simulink model "Assingment1_3K04_Part1_Group_7"  (R2017b)
settings: Solver=FixedStepAuto  StartTime=0.0  StopTime=3  FixedStep=1e-3  RelTol=1e-3  EnableMultiTasking=on
undefined symbols (not defined in the file): D10, D11, D12, D13, D2, D3, D4, D5, D6, D7, D8, D9, PTA0, PTA1, PTA2, PTB23, PTB9, PTC2, PTC3, PTC4, PTD0, PTD1, PTD2, PTD3
libraries: frdmk64flib x14
settings Model: ExtModeTrigDuration=5  Creator=howla_000  LastModifiedBy=gagiche
settings DataIOCC: LimitDataPoints=on  SaveFormat=Array
settings OptimizationCC: PassReuseOutputArgsAs=Individual arguments  MaxStackSize=64
settings DebuggingCC: UnderspecifiedInitializationDetection=Classic  MergeDetectMultiDrivingBlocksExec=none  SolverPrmCheckMsg=warning  ParameterTunabilityLossMsg=error  StateNameClashWarn=warning  SFUnexpectedBacktrackingDiag=warning  SFNoUnconditionalDefaultTransitionDiag=warning  SFExecutionAtInitializationDiag=none
settings HardwareCC: ProdBitPerPointer=32  ProdBitPerSizeT=32  ProdBitPerPtrDiffT=32  ProdLargestAtomicInteger=Long  ProdLargestAtomicFloat=Double  ProdWordSize=32  ProdHWDeviceType=ARM Compatible->ARM Cortex
settings ModelReferenceCC: PropagateSignalLabelsOutOfModel=off
settings SFSimCC: MATLABDynamicMemAlloc=off
settings RTWCC: SystemTargetFile=ert.tlc  HardwareBoard=NXP FRDM-K64F  TemplateMakefile=ert_default_tmf  GenerateReport=on  Toolchain=GNU Tools for ARM Embedded Processors  IncludeHyperlinkInReport=on  LaunchReport=on  GenerateTraceInfo=on  GenerateTraceReport=on  GenerateTraceReportSl=on  GenerateTraceReportSf=on  GenerateTraceReportEml=on
settings CodeAppCC: ForceParamTrailComments=on  IgnoreCustomStorageClasses=off  OperatorAnnotations=on  SimulinkDataObjDesc=on  SFDataObjDesc=on  InsertBlockDesc=on
settings ConfigComp: CovMetricSettings=dw  CovHtmlReporting=on  CovSaveCumulativeToWorkspaceVar=on  CovSaveSingleToWorkspaceVar=on  CovExternalEMLEnable=off
settings SimscapeCC: SimscapeNormalizeSystem=off

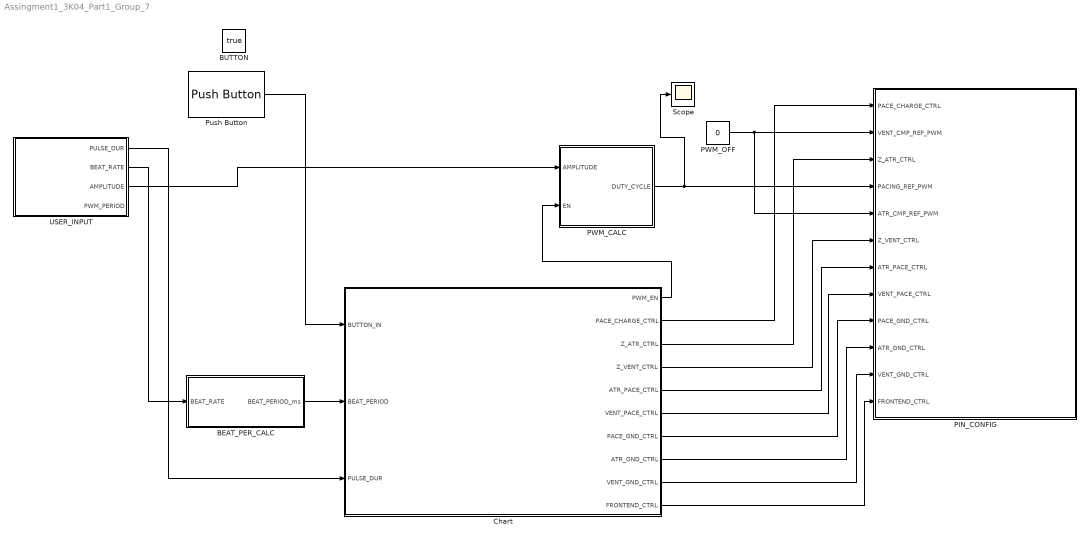
== system Assingment1_3K04_Part1_Group_7 ==
  BEAT_PER_CALC : Subsystem
  BUTTON : Constant  Value=true  OutDataTypeStr=boolean
  Chart : Stateflow chart  TreatAsAtomicUnit=on
  "PIN_CONFIG " : Subsystem
  PWM_CALC : Subsystem
  PWM_OFF : Constant  Value=0  OutDataTypeStr=uint16
  Push Button : frdmk64flib/Push Button  Whichswitch=SW2  SampleTime1=-1
      settings: SourceProductName=Simulink Coder Support Package for NXP FRDM-K64F Board
  Scope : Scope
  USER_INPUT : Subsystem
  wires:
  USER_INPUT/3("AMPLITUDE ") -> PWM_CALC/1(AMPLITUDE)
  PWM_CALC/1(DUTY_CYCLE) -> Scope/1, "PIN_CONFIG "/4(PACING_REF_PWM)
  Chart/2(PACE_CHARGE_CTRL) -> "PIN_CONFIG "/1(PACE_CHARGE_CTRL)
  Chart/3(Z_ATR_CTRL) -> "PIN_CONFIG "/3(Z_ATR_CTRL)
  Chart/5(ATR_PACE_CTRL) -> "PIN_CONFIG "/7(ATR_PACE_CTRL)
  Chart/4(Z_VENT_CTRL) -> "PIN_CONFIG "/6(Z_VENT_CTRL)
  Chart/6(VENT_PACE_CTRL) -> "PIN_CONFIG "/8(VENT_PACE_CTRL)
  Chart/7(PACE_GND_CTRL) -> "PIN_CONFIG "/9(PACE_GND_CTRL)
  Chart/8(ATR_GND_CTRL) -> "PIN_CONFIG "/10(ATR_GND_CTRL)
  Chart/9(VENT_GND_CTRL) -> "PIN_CONFIG "/11(VENT_GND_CTRL)
  Chart/10(FRONTEND_CTRL) -> "PIN_CONFIG "/12(FRONTEND_CTRL)
  USER_INPUT/1("PULSE_DUR ") -> Chart/3(PULSE_DUR)
  BEAT_PER_CALC/1(BEAT_PERIOD_ms) -> Chart/2(BEAT_PERIOD)
  USER_INPUT/2("BEAT_RATE ") -> BEAT_PER_CALC/1(BEAT_RATE)
  PWM_OFF/1 -> "PIN_CONFIG "/5(ATR_CMP_REF_PWM), "PIN_CONFIG "/2(VENT_CMP_REF_PWM)
  Push Button/1 -> Chart/1(BUTTON_IN)
  Chart/1(PWM_EN) -> PWM_CALC/2(EN)

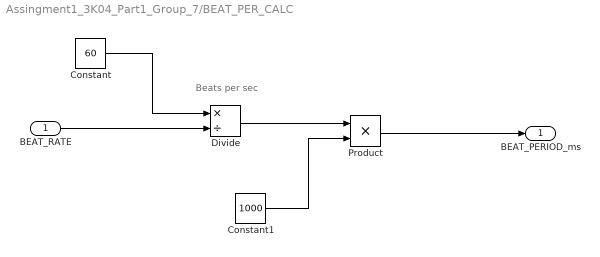
== system Assingment1_3K04_Part1_Group_7/BEAT_PER_CALC ==
  note: Beats per sec
  BEAT_RATE : Inport
  Constant : Constant  Value=60  OutDataTypeStr=double
  Constant1 : Constant  Value=1000  OutDataTypeStr=uint32
  Divide : Product  Inputs=*/  OutDataTypeStr=double
  Product : Product  OutDataTypeStr=double
  BEAT_PERIOD_ms : Outport  OutDataTypeStr=double
  wires:
  Divide/1 -> Product/1
  Product/1 -> BEAT_PERIOD_ms/1
  Constant1/1 -> Product/2
  BEAT_RATE/1 -> Divide/2
  Constant/1 -> Divide/1

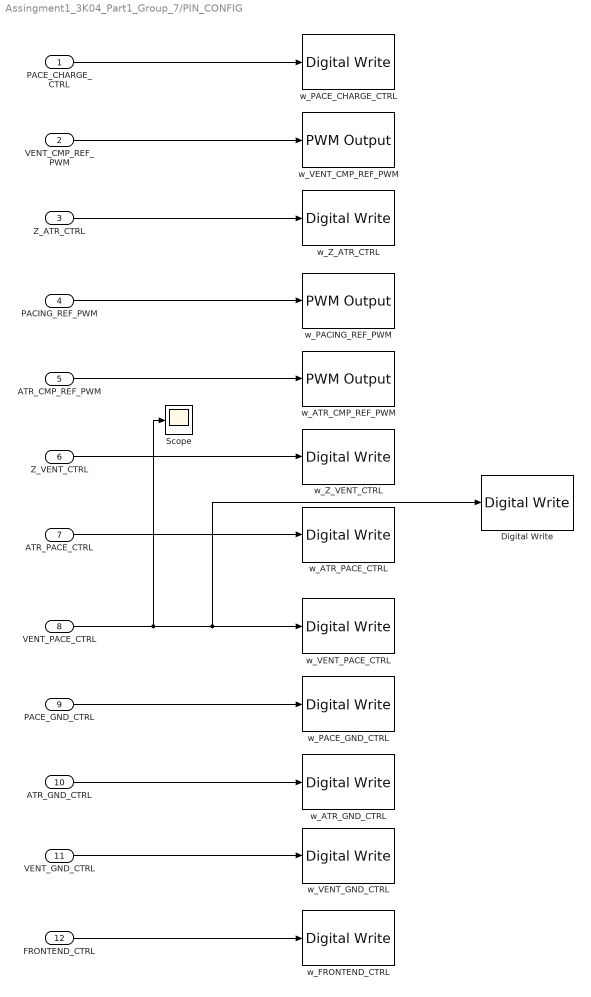
== system Assingment1_3K04_Part1_Group_7/PIN_CONFIG  ==
  PACE_CHARGE_CTRL : Inport
  VENT_CMP_REF_PWM : Inport  Port=2
  Z_ATR_CTRL : Inport  Port=3
  PACING_REF_PWM : Inport  Port=4
  ATR_CMP_REF_PWM : Inport  Port=5
  Z_VENT_CTRL : Inport  Port=6
  ATR_PACE_CTRL : Inport  Port=7
  VENT_PACE_CTRL : Inport  Port=8
  PACE_GND_CTRL : Inport  Port=9
  ATR_GND_CTRL : Inport  Port=10
  VENT_GND_CTRL : Inport  Port=11
  FRONTEND_CTRL : Inport  Port=12
  Digital Write : frdmk64flib/Digital Write  Whichpin=BLUE_LED
      settings: SourceProductName=Simulink Coder Support Package for NXP FRDM-K64F Board
  Scope : Scope
  w_ATR_CMP_REF_PWM : frdmk64flib/PWM Output  Whichpin=PTC2 (D6)  InitialFrequency=1000  InitialDutyCycle=0
      settings: SourceProductName=Simulink Coder Support Package for NXP FRDM-K64F Board
  w_ATR_GND_CTRL : frdmk64flib/Digital Write  Whichpin=PTD2 (D11)
      settings: SourceProductName=Simulink Coder Support Package for NXP FRDM-K64F Board
  w_ATR_PACE_CTRL : frdmk64flib/Digital Write  Whichpin=PTA0 (D8)
      settings: SourceProductName=Simulink Coder Support Package for NXP FRDM-K64F Board
  w_FRONTEND_CTRL : frdmk64flib/Digital Write  Whichpin=PTD1 (D13)
      settings: SourceProductName=Simulink Coder Support Package for NXP FRDM-K64F Board
  w_PACE_CHARGE_CTRL : frdmk64flib/Digital Write  Whichpin=PTB9 (D2)
      settings: SourceProductName=Simulink Coder Support Package for NXP FRDM-K64F Board
  w_PACE_GND_CTRL : frdmk64flib/Digital Write  Whichpin=PTD0 (D10)
      settings: SourceProductName=Simulink Coder Support Package for NXP FRDM-K64F Board
  w_PACING_REF_PWM : frdmk64flib/PWM Output  Whichpin=PTA2 (D5)  InitialFrequency=1000  InitialDutyCycle=0
      settings: SourceProductName=Simulink Coder Support Package for NXP FRDM-K64F Board
  w_VENT_CMP_REF_PWM : frdmk64flib/PWM Output  Whichpin=PTA1 (D3)  InitialFrequency=1000  InitialDutyCycle=0
      settings: SourceProductName=Simulink Coder Support Package for NXP FRDM-K64F Board
  w_VENT_GND_CTRL : frdmk64flib/Digital Write  Whichpin=PTD3 (D12)
      settings: SourceProductName=Simulink Coder Support Package for NXP FRDM-K64F Board
  w_VENT_PACE_CTRL : frdmk64flib/Digital Write  Whichpin=PTC4 (D9)
      settings: SourceProductName=Simulink Coder Support Package for NXP FRDM-K64F Board
  w_Z_ATR_CTRL : frdmk64flib/Digital Write  Whichpin=PTB23 (D4)
      settings: SourceProductName=Simulink Coder Support Package for NXP FRDM-K64F Board
  w_Z_VENT_CTRL : frdmk64flib/Digital Write  Whichpin=PTC3 (D7)
      settings: SourceProductName=Simulink Coder Support Package for NXP FRDM-K64F Board
  wires:
  PACE_CHARGE_CTRL/1 -> w_PACE_CHARGE_CTRL/1
  VENT_CMP_REF_PWM/1 -> w_VENT_CMP_REF_PWM/1
  Z_ATR_CTRL/1 -> w_Z_ATR_CTRL/1
  PACING_REF_PWM/1 -> w_PACING_REF_PWM/1
  ATR_CMP_REF_PWM/1 -> w_ATR_CMP_REF_PWM/1
  Z_VENT_CTRL/1 -> w_Z_VENT_CTRL/1
  ATR_PACE_CTRL/1 -> w_ATR_PACE_CTRL/1
  VENT_PACE_CTRL/1 -> Scope/1, Digital Write/1, w_VENT_PACE_CTRL/1
  PACE_GND_CTRL/1 -> w_PACE_GND_CTRL/1
  ATR_GND_CTRL/1 -> w_ATR_GND_CTRL/1
  VENT_GND_CTRL/1 -> w_VENT_GND_CTRL/1
  FRONTEND_CTRL/1 -> w_FRONTEND_CTRL/1

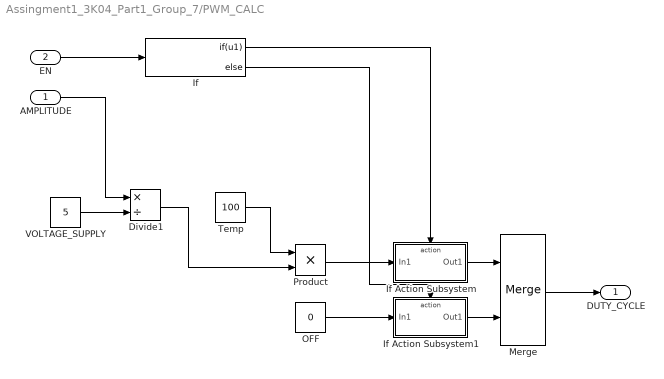
== system Assingment1_3K04_Part1_Group_7/PWM_CALC ==
  AMPLITUDE : Inport  OutDataTypeStr=double
  EN : Inport  Port=2  OutDataTypeStr=boolean
  Divide1 : Product  Inputs=*/  OutDataTypeStr=double
  If : If  IfExpression=u1
  If Action Subsystem : Subsystem  TreatAsAtomicUnit=on
  If Action Subsystem1 : Subsystem  TreatAsAtomicUnit=on
  Merge : Merge
  OFF : Constant  Value=0  OutDataTypeStr=uint32
  Product : Product  OutDataTypeStr=uint32
  "Temp " : Constant  Value=100  OutDataTypeStr=double
  "VOLTAGE_SUPPLY " : Constant  Value=5  OutDataTypeStr=double
  DUTY_CYCLE : Outport  OutDataTypeStr=uint32  LockScale=on
  wires:
  "VOLTAGE_SUPPLY "/1 -> Divide1/2
  "Temp "/1 -> Product/1
  EN/1 -> If/1
  Merge/1 -> DUTY_CYCLE/1
  If Action Subsystem/1(Out1) -> Merge/1
  If Action Subsystem1/1(Out1) -> Merge/2
  Product/1 -> If Action Subsystem/1(In1)
  If/1 -> If Action Subsystem/Action
  If/2 -> If Action Subsystem1/Action
  OFF/1 -> If Action Subsystem1/1(In1)
  AMPLITUDE/1 -> Divide1/1
  Divide1/1 -> Product/2

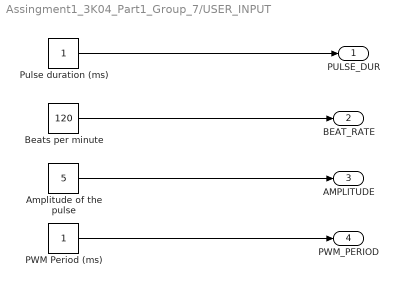
== system Assingment1_3K04_Part1_Group_7/USER_INPUT ==
  Amplitude of the pulse : Constant  Value=5
  Beats per minute : Constant  Value=120
  PWM Period (ms) : Constant  OutDataTypeStr=uint16
  Pulse duration (ms) : Constant  OutDataTypeStr=double
  "PULSE_DUR " : Outport  OutDataTypeStr=double
  "BEAT_RATE " : Outport  Port=2
  "AMPLITUDE " : Outport  Port=3
  PWM_PERIOD : Outport  Port=4
  wires:
  Pulse duration (ms)/1 -> "PULSE_DUR "/1
  Beats per minute/1 -> "BEAT_RATE "/1
  Amplitude of the pulse/1 -> "AMPLITUDE "/1
  PWM Period (ms)/1 -> PWM_PERIOD/1

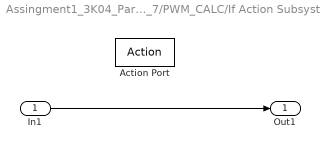
== system Assingment1_3K04_Part1_Group_7/PWM_CALC/If Action Subsystem ==
  In1 : Inport
  Action Port : ActionPort  ActionType=then
  Out1 : Outport
  wires:
  In1/1 -> Out1/1

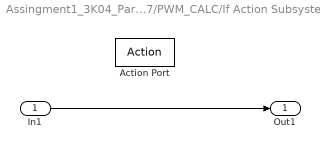
== system Assingment1_3K04_Part1_Group_7/PWM_CALC/If Action Subsystem1 ==
  In1 : Inport
  Action Port : ActionPort  ActionType=else
  Out1 : Outport
  wires:
  In1/1 -> Out1/1

== stateflow chart Assingment1_3K04_Part1_Group_7/Chart ==
  state CHARGE
    entry:
    PACE_GND_CTRL = 1;
    VENT_PACE_CTRL = 0;
    Z_ATR_CTRL = 0;
    Z_VENT_CTRL = 0;
    ATR_PACE_CTRL = 0;
    ATR_GND_CTRL = 0;
    VENT_GND_CTRL = 1;
    FRONTEND_CTRL = 0;
    PWM_EN = true;
    PACE_CHARGE_CTRL = 1;
  state DISCHARGE
    entry:
    if (BUTTON_IN == false)
    PACE_CHARGE_CTRL = 0;
    PACE_GND_CTRL = 1;
    ATR_PACE_CTRL = 0;
    ATR_GND_CTRL = 0;
    Z_ATR_CTRL = 0;
    Z_VENT_CTRL = 0;
    VENT_GND_CTRL = 0;
    VENT_PACE_CTRL = 1;
    FRONTEND_CTRL = 0;
    end
  (default) -> CHARGE
  CHARGE -> DISCHARGE : after(BEAT_PERIOD - PULSE_DUR, msec)
  DISCHARGE -> CHARGE : after(PULSE_DUR, msec)
  data: PWM_EN output; BUTTON_IN input boolean; BEAT_PERIOD input double; PULSE_DUR input double; PACE_CHARGE_CTRL output; Z_ATR_CTRL output; Z_VENT_CTRL output; ATR_PACE_CTRL output; VENT_PACE_CTRL output; PACE_GND_CTRL output; ATR_GND_CTRL output; VENT_GND_CTRL output; FRONTEND_CTRL output
